simulink model "FullyConnectedMMG"  (R2020b)
settings: Solver=ode3  StartTime=0.0  StopTime=TimeS  FixedStep=Ts  RelTol=1e-3
values from neighbouring files (symbols this model uses):
  fr = 60    [MMG_Parameters.m]
  Lgs = 600e-6    (= 0.0006)    [MMG_Parameters.m]
  MaxWind = 18    [MMG_Parameters.m]
  MicroVol = 575    [MMG_Parameters.m]
  MinWind = 3    [MMG_Parameters.m]
  NomVol = 600    [MMG_Parameters.m]
  NomWind = 10    [MMG_Parameters.m]
  Pnombb = 400    [MMG_Parameters.m]
  PnomDG = 150e3    (= 150000)    [MMG_Parameters.m]
  PnomWT = 400e3    (= 400000)    [MMG_Parameters.m]
  Rgs = 20e-6    (= 2e-05)    [MMG_Parameters.m]
  RtCapM1 = (5.1)*1e-1    (= 0.51)    [MMG_Parameters.m]
  RtCapM2 = (5.1)*1e-1    (= 0.51)    [MMG_Parameters.m]
  SOC = [70,80,75,65]    [MMG_Parameters.m]
  Ts = 8e-4    (= 0.0008)    [MMG_Parameters.m]    (also in SolveMONO.m = 0.005)
  Vgrid = 25e3    (= 25000)    [MMG_Parameters.m]
  VMic = 575    [MMG_Parameters.m]
  Vs = 120e3    (= 120000)    [MMG_Parameters.m]
undefined symbols (not defined in the file or in its folder): DiscIntNeverNeededParam
libraries: powerlib x64, simulink x24, powerlib_meascontrol x16
(part 4 of 5)

== matlab function FullyConnectedMMG/Subsystem/Subsystem2/MATLAB Function ==
  settings: updateMethod=DISCRETE
  data: Hour input; xInput input; outGrid output; shMGs output; recMGs output; Flag output
 function [outGrid,shMGs,recMGs,Flag] = States(Hour,xInput)
%% Parameters For Objective Function %%
%%%%%%%%%%%%%%%%%%%%%%%%%%%%%%%%%%%%%%%
% The objective function in the second layer is established to improve costs in the entire MMG system -%
% The CEMS in this layer aims to minimize costs caused by power exchanged between MGs into 
% the MMG system and as well as power losses caused by transactions % 

% ********************** %
% The Objective Function %
% ********************** %
% f =  sum(Cg*(Pm^{Ug}(t) + Pm^{lossg}(t)) + Cexc(Pmj^{exc}(t) + Pmj^{lossMG}(t))

% Note: It is important to note that in this case we only need one RNN
% to solve the single-objective optimization problem. 

%%%%%%%%%%%%%%%%%%%%%%%%%%%%%%%%%%%%%%%%%%%%%%%
%% Call The Function That Containts The DPNN %%
%%%%%%%%%%%%%%%%%%%%%%%%%%%%%%%%%%%%%%%%%%%%%%%
% In this case, xInput are the references for power exchanged between the
% MGs and the grid established in the first layer by the NEMS  
% Hour, is the respective time slot.

numMGs = length(xInput);                        	% Number of MGs within the MMG system

%- Define the dimension of output variables -%
outGrid = zeros(numMGs,1); shMGs = zeros(numMGs,1);  recMGs = zeros(numMGs,1);  oErr = zeros(numMGs,1);  Flag = 0;

%- Call the main function to perform the optimization in the CEMS -%
[outGrid,shMGs,recMGs,oErr,Flag] = Optimization(xInput, Hour, numMGs);

%- Print information about optimization -%
    nMGs = (1:numMGs);
    status = cell(numMGs,1);
    
    for k=1:length(nMGs)
        if xInput(k) < 0
            status{k} = 'Surplus';
        else
            status{k} = 'Deficit';
        end
    end
    
    wkW = 1e-3;
    fprintf(' ------------------------------------------------- \n || Info about optimization in the second layer || \n ------------------------------------------------- \n');
    Table2 = table((wkW)*xInput,status,(wkW)*outGrid,(wkW)*shMGs,(wkW)*recMGs,oErr,...
                'VariableNames',{'| Ener. net |','| Status |','| Ener. Grid |','| Ener. shared |','|Ener. received |','| Error |' },'RowName',{'|| MG1 ||','|| MG2 ||'})
    fprintf('\n|| -o-o-o-o-o-o-o-o-o-o-o-o-o-o-o-o-o-o-o-o-o-o-o-o-o-o-o-o-o-o-o-o-o-o-o-o-o-o-o-o-o-o-o-o-o-o-o-o-o-o-o-o-o-o-o-o-o-o-o-o-o-o-o-o-o-o-o-o-o-o-o-o-o-o-o-o-o-o-o-o-o- ||');    
    
    %formatSpec = '|| MG %1.0f || Status: %s, EnergyNet: %4.2f, Grid: %4.2f, Sharing: %4.2f, Receiving: %4.2f, Error: %3.2f \n';
    %fprintf(' --------------------------------------- \n | Info of optimization in the second layer | \n --------------------------------------- \n');
    %for k=1:length(nMGs)
    %    if xInput(k) < 0
    %        status = "Sur";
    %    else
    %        status = "Def";
    %    end
    %    fprintf(formatSpec,nMGs(k),status,xInput(k),outGrid(k),shMGs(k),recMGs(k),oErr(k));
    %end
% fprintf('\n|| -o-o-o-o-o-o-o-o-o-o-o-o-o-o-o-o-o-o-o-o-o-o-o-o-o-o-o-o-o-o-o-o-o-o-o-o-o-o-o-o-o-o-o-o-o-o-o-o-o-o-o-o-o-o-o-o-o-o-o-o-o-o-o-o-o-o-o-o-o-o-o-o-o-o-o-o-o-o-o-o-o- ||');    

end

% %%%%%%%%%%%%%%%%%%%% %
%- Auxiliar Functions -%
% %%%%%%%%%%%%%%%%%%%% %

% **************************** %
%- Main Optimization Function -%
% **************************** %
function [oGrid,shMGs,recMGs,oErr,Flag] = Optimization(eInp,hr,nMG)
%%%%%%%%%%%%%%%%%
%% Some notes: %%
%%%%%%%%%%%%%%%%%
%%%%%%%%%%%%%%%%%%%%%%%%%%%%%%%%%%%%%%%%%%%%%%%%%%%%
%- This function will output two vectors, where:   %
%  oGrid = [Energy imp/exp from/to grid in MG_m];  %


%  oMGs = [Energy imp/exp from/to MGj in MG_m];    %
%  For m = 1,.., M.                                %

%  oGrid and oMGs are vectors of dimension 
% [nMG x 1], respectively. -%
%%%%%%%%%%%%%%%%%%%%%%%%%%%%%%%%%%%%%%%%%%%%%%%%%%%%

%- eInp = Energy statuts (Surplus/deficit energy in each MG) -%
    Auxv = zeros(nMG,1);                    % Auxiliar vector to check the status of energy in MGs (deficit/surplus)
    for i=1:nMG
        if eInp(i) < 0
            Auxv(i,1) = 1;                  % "1" Means that there exists surplus energy
        else
            Auxv(i,1) = 0;                 	% "0" Means that there exists deficit energy
        end
    end
 
    surVect = find(Auxv);                 	% Indixes of MGs with surplus energy 
    lenSur = length(surVect);            	% Number of MGs with surplus energy
    
    defVect = find(~Auxv);                 	% Indixes of MGs with deficit energy
    lenDef = length(defVect);            	% Number of MGs with deficit energy
    
%%%%%%%%%%%%%%%%%%%%%%%%%%%%%%%%%%%%%%%%%%%%%%%%%%%%%%%%%%%%%%%    
%- Perform theans Global Optimization If There Exist Conditions -%
%%%%%%%%%%%%%%%%%%%%%%%%%%%%%%%%%%%%%%%%%%%%%%%%%%%%%%%%%%%%%%%
    EnableGO = 0;                                   % Enable Global Optimization (1= Enable, 0 = Disable)
    %- Check that there exist one MG with surplus and 
    % other one with deficit energy.
    if (lenSur ~= 0 && lenDef ~= 0 && EnableGO ==1)       
    % Use neural netowrk function to perform the optimization %
        [outX,oErr] = NNfunc(surVect,defVect,eInp,nMG,hr);       
        oGrid = outX(:,1);
        shMGs = outX(:,2);
        recMGs = outX(:,3);
    else
        % Not perform the optimization because the conditions are not satisfied.
        oGrid = eInp;                                       
        shMGs = zeros(nMG,1);                               
        recMGs = zeros(nMG,1);
        
        oErr = (11.11)*ones(nMG,1);
    end   
    Flag = hr + 1;
end

% ************************* %
%- Neural Network Function -%
% ************************* %
function [xOpt,Error] = NNfunc(surVec,defVec,xEn,nMG,hour)
    %- Required parameters for neural networks -%
    nVar = 2;                                           % Number of desicion variables
    Ts = 5e-3;                                          % Step size for the solver
    Lamb = 6;                                           % Rate of convergence for the neural network (Workin: Lamb = ??);
    ite = 2500;              % 20000;                    % Max number of iterations to integrate the differential equations
    
    xOpt = [xEn,zeros(nMG,2)];                          % Establish the output vector
    
    %- Bounds for exchanged power in the MMG system -%     
    Mingrid = 0;                                        % (Kw/h)   Max power exported to the grid 
    Minsh = 0;                                          % (Kw/h)   Min power shared by an MG with surplus power
    
    %- Auxiliar variables -%
    shPower = zeros(length(surVec),nVar);               % Auxiliar vector to save the relation between MGs exchanging energy
    auxOpt = zeros(length(surVec),nVar);                % Auxiliar vector to save optimal values 
    
    Error = (11.11)*ones(nMG,1);                                % Auxiliar vector to observe the error produced during optimization
       
    % Maxgrid = (1e4)*150;                             	% kW/h   Max power imported from the grid
    
    %%%%%%%%%%%%%%%%%%%%%%%%%%%%%%%
    %- Main Loop of optimization -%
    %%%%%%%%%%%%%%%%%%%%%%%%%%%%%%%
    %- Select an MG with surplus energy and perform an optimization with
    % each MG with deficit of power. 
    for i=1:length(surVec)                         
        vecX = zeros(length(defVec),2);               	% Auxiliar vector of solutions
        costX = zeros(length(defVec),1);             	% Auxiliar vector of costs
        
        for j=1:length(defVec)
         	Maxgrid = abs(xEn(surVec(i)));          	% The Max power that can inject to the grid is the 
                                                        % total of surplus energy 
            
            Maxsh_rec = min(Maxgrid,xEn(defVec(j)));    % The max power received by a MG will be the min 
                                                        % between the surplus power of MGi and deficit power of MGj
            
            %- Establish the upper and lower bounds for decision variables -%                                            
            UpB = [Maxgrid;Maxsh_rec];                  % Upper bound
            LowB = [Mingrid;Minsh];                     % Lower bound
            % -------------------------------------------------------------- %
            %- Call objective function f(x) and its derivative in this layer %
            % ---------------------------------------------------------------% 
            [Func,gFunc] = ObjFunct(xEn,i,j,hour);   
            %- Variables used for the equality constraint -%
            A = [1,1];                                  % We have only two variable decisions:
                                                        % Energy shared
                                                        % with the grid and the energy shared with other MG
                                                        
            b = abs(xEn(surVec(i)));                    % In this case, we consider the energy shared with the grid 
                                                        % and with other MG j mustbe the same of surplus energy in MG i 

           	%- Initial value for decision variable x -%
          	Ic = abs(UpB(1))/2;
            % Iincr = 20;
            Iincr = abs(UpB(1))/15;
            
            x = [Ic-Iincr;Ic+Iincr];
            
            % x = [unifrnd(Mingrid,Maxgrid);unifrnd(Minsh,Maxsh_rec)]; 
            
            %- Check these conditions (Maybe are not necessary) -%
            counter = 1;
            condConv = true;
            
            %%%%%%%%%%%%%%%%%%%%%%%%%%%%%%%%%%
            %- Main loop of neural networks -%
            %%%%%%%%%%%%%%%%%%%%%%%%%%%%%%%%%%                     
            while condConv
                %%%%%%%%%%%%%%%%%%%%%%%%%%%%%%%%%%%%%%%%%%%%
                %- Structure of recurrent neural networks -%
                %%%%%%%%%%%%%%%%%%%%%%%%%%%%%%%%%%%%%%%%%%%%
                % ************************* %
              	% Structure of our approach %
              	% ************************* %
                sig = -(0.5)*ones(1,1);                             % Initial values for sigma 
                Px = zeros(length(x),1);                            % Auxiliar variable for the projection
                %- Gains used by the activation functions y and z %
                if hour == 14
                    k2 = 100;     % Original values
                    k1 = 85.5;    % Original values    
                elseif hour == 15
                    k2 = 100;     % Original values
                    k1 = 205.5;    % Original values    
                else
                    k2 = 100;
                    k1 = 65.5;  
                end

                %- Integrate the differential equations of neural networks -% 
                for it=1:ite                           	              
                    % Finite-Time Stabilizer (Lagrange Multiplier y)%
                    y = Stabilizer(UpB,LowB,k2,x);
                    % Finite-time sliding mode operator (Lagrange Multiplier z) %
                    z = SMOperator(UpB,LowB,k1,x,sig);    
                    %- Apply the projection -%
                  	for n = 1:length(x)
                        Px(n,1) = Pr(LowB(n),UpB(n),x(n));          	 
                    end
                    %- Dynamic for Recurrent Neural Network -%
                    dx = Lamb*(-gFunc(Px) + Px - x + A'*z + y);
                    %- Dynamic for variable related with the sliding surface -%
                    dsig = Lamb*(-A*gFunc(Px) + A*Px - A*x + A*A'*z + A*y); 
                    %- Integration of differential equations related to neural networks -%
                    tspan = [0 Ts];
                    [~,xout] = ode23(@(tx,xout) dx, tspan, x);
                    [~,sigout] = ode23(@(tz,sigout) dsig, tspan, sig);
                    %- Output variables of ODE -%
                    x = xout(end,:)';
                    sig = sigout(end,:);
                    %- Check the error obtained -%
                    if abs(sum(x) - b) < 0.5                %Work: 0.3
                        condConv = false;
                        break;
                    end
                end
             	counter = counter + 1;
                if counter > 4
                    condConv = false;
                end               
            end 
            vecX(j,:) = x';
            costX(j) = Func(x); 
        end
        
        % Select Solutions With Best Values (Minor Costs) %
        [~,Index] = min(costX);
        % Save The Relation Between There Exists a Exchanged Power
        shPower(i,:) = [surVec(i),defVec(Index)];
        % Save Optimal Values %
        auxOpt(i,:) = vecX(Index,:);
        % Determinate Errors;
        Error(surVec(i)) = abs(sum(auxOpt(i,:)) - abs(xEn(surVec(i))));
        % Modify Output Vector Of Exchanged Power %
        xOpt(surVec(i),1:2) = -vecX(Index,:);
        % xOpt(surVec(i),3) = 0;
        xOpt(defVec(Index),1) = xOpt(defVec(Index),1) - vecX(Index,2);
        %xOpt(defVec(Index),2) = 0;
        xOpt(defVec(Index),3) = vecX(Index,2);
        
        % Delete Used Indexes %
        % surVec(i) = [];
        defVec(Index) = [];
        if isempty(defVec)
            break;
        end
    end
end
   
% ******************** %
%- Objective Function -%
% ******************** %
function [Func,gFunc] = ObjFunct(eneVec,i,j,hr)
    %- Establish the cost of grid energy according the hour of the day -%
    peak = [(8:11),(16:21)];                % (Hr) Period of time for peak tariff category 
    plain = (12:15);                        % (Hr) Period of time for plain tariff category
    %   valley = [(1:7),(22:24)];          	% (Hr) Period of time for valley tariff category
    if ismember(hr,peak)
        % Peak tariff %
        Cgpur = 0.21;   %0.17               % (USD/Kwh) Cost of purchasing energy from the grid 
        Cgsell = 0.11;                      % (USD/kWh) Cost of selling energy to the grid
    elseif ismember(hr,plain)
       	% Plain tariff %
        Cgpur = 0.14;                       % (USD/Kwh) Cost of purchasing energy from the grid 
        Cgsell = 0.051;                     % (USD/kWh) Cost of selling energy to the grid
    else
        % Valley tariff % 
        Cgpur = 0.062;                      % (USD/Kwh) Cost of purchasing energy from the grid
        Cgsell = 0.039;                     % (USD/kWh) Cost of selling energy to the grid
    end  
    %- Check if energy will be purchased/sold from/to the grid -%
    if eneVec < 0   
        % Cg = Cgpur;                       % The MG is purchasing energy from the grid   
        sell = 0;
        Pur = 1;
    else
        %Cg = Cgsell;                       % The MG is sellig energy to the grid
        sell = 1;
        Pur = 0;
    end
    % Volatage in transmission lines %
    UMG = 575;                              % (V) voltage of the distribution lines in the MMG system
    % Cheeeeeeeeeeeeeeeeeeeeeeeeeeck this voltage %
    Ugrid = 575;                            % (V) voltage of the distribution lines between the MGs and the grid
    % AuxRgrid = [1.55,1.75,1.875,1.7];
    AuxRgrid = [3.1,3.15,3.705,2.5875];
    Rgrid = AuxRgrid(i);                    % (Ohms) Resistance of the distribution lines between MG i and the grid 
    %- Resistance in transmission lines among the MGs within the MMG system -%
    AuxRMGs = [ 1,   0.4,  0.1,  0.08;
            0.4,  1,   0.06, 0.05;
            0.1,  0.06, 1,   0.02;
            0.08, 0.05, 0.02, 1];
        
    RMGs = AuxRMGs(i,j);                    % Select the resistence of transmission lines between MGi and MGj
    %- Coeffcients costs (of sharing-receiving power among MGs) -%
    Csh = 0.005;        % 0.01;           	% (USD/Kwh) Cost of share (sell) energy with other MG
    Crec = 0.005;       % 0.01;            	% (USD/Kwh) Cost Of receieve (purchase) energy from other MG
    %%%%%%%%%%%%%%%%%%%%%%%%%%%%%%%%%%%%%%
    %% Objective function (in the CEMS) %%
    %%%%%%%%%%%%%%%%%%%%%%%%%%%%%%%%%%%%%%
    %- Objective Function -%
    Plossgrid = @(x) (x(1)^2)*(Rgrid/(Ugrid^2));
    PlossMG =   @(x) (x(2)^2)*(RMGs/(UMG^2));
    
    Func =  @(x) Pur*Cgpur*x(1) + sell*Cgsell*x(1) + Pur*Cgpur*Plossgrid(x) + sell*Cgsell*Plossgrid(x)...
                +Pur*Crec*x(2) + sell*Csh*x(2) + sell*Csh*PlossMG(x) + Pur*Crec*PlossMG(x);
    
    %- Gradient of objective optimization function -%
    gFunc = @(x) [Pur*Cgpur + sell*Cgsell + Pur*Cgpur*2*x(1)*(Rgrid/(Ugrid^2)) + sell*Cgsell*2*x(1)*(Rgrid/(Ugrid^2));
                  sell*Csh + Pur*Crec + sell*Csh*2*x(2)*(RMGs/(UMG^2)) + sell*Cgsell*2*x(2)*(RMGs/(UMG^2))];   

    % Check if the output values of these functions coincide with the above functions %
              
    % Func1 =  @(x) Pur*Cgpur*x(1) + sell*Cgsell*x(1) + Pur*Cgpur*(x(1)^2)*(Rgrid/(Ugrid^2)) + sell*Cgsell*(x(1)^2)*(Rgrid/(Ugrid^2))...
    %            + sell*Csh*x(2) + Pur*Crec*x(2) + sell*Csh*(x(2)^2)*(RMGs/(UMG^2)) + Pur*Crec*(x(2)^2)*(RMGs/(UMG^2));
              
    % gFunc = @(x) [Pur*Cgpur + sell*Cgsell + Pur*Cgpur*2*x(1)*(Rgrid/(Ugrid^2)) + sell*Cgsell*2*x(1)*(Rgrid/(Ugrid^2));
    %              sell*Csh + Pur*Crec + sell*Csh*2*x(2)*(RMGs/(UMG^2)) + sell*Cgsell*2*x(2)*(RMGs/(UMG^2))];                 

%{
    % Objective Function %
    Func =  @(x) fExp*fEimp*Cgpur*x(1) + fExp*fEimp*Cgsell*x(1) + Closs*(x(1)^2)*(Rgrid/(Ugrid^2))...
                + fExp*fEimp*Csh*x(2) + fExp*fEimp*Crec*x(2) + Closs*(x(2)^2)*(RMGs/(UMG^2));
    
    %- Gradient of Objective Optimization Function %
    gFunc = @(x) [fExp*fEimp*Cgpur + fExp*fEimp*Cgsell + 2*Closs*x(1)*(Rgrid/(Ugrid^2));
                  fExp*fEimp*Csh + fExp*fEimp*Crec + 2*Closs*x(2)*(RMGs/(UMG^2))];
%}              
end

% ********************************** %
%- Function to apply the projection -%
% ********************************** %
function y = Pr(Lbx, Ubx, xin)
    y = 0;
    idx1 = xin <= Lbx;
    y(idx1) = Lbx;
    idx2 = xin >= Ubx;
    y(idx2) = Ubx;
    y(~(idx1 | idx2)) = xin;
end

% ********************************************************************** %
%- Finite Time Stabilizer Function (Used to reach the bound constraints)-%
% ********************************************************************** %
function Outy = Stabilizer(Ubx,Lbx,k,eta)
    % Auxiliar variables %
    Outy = zeros(length(eta),1); 
    xl = norm(eta - Lbx);  
    xh = norm(eta - Ubx);
    % Select Case %
    for i = 1:length(eta)
        if eta(i) < Lbx(i)          % x < l
            Outy(i,1) = -k*((eta(i) - Lbx(i))/xl);
        elseif  eta(i) > Ubx(i)     % x > h
            Outy(i,1) = -k*((eta(i) - Ubx(i))/xh);
        else
            Outy(i,1) = 0;
        end
    end
end

% *************************************************************** %
%- Finite time sliding mode operator:                             % 
% (Used to reach the sliding surface inside the bound constraints %
% *************************************************************** %
function Outz = SMOperator(Ubx,Lbx,k,eta,sig)
  	% Auxiliar variables %
    % Outz = zeros(length(sig),1);    
    % Check Bounds and Select Case %
    if eta > Ubx           
        Outz = zeros(length(sig),1);
    elseif eta < Lbx
        Outz = zeros(length(sig),1);
    else
        Outz = -k*(sig/norm(sig));     % l < x < h
    end
        
end

% **************** %
%- Delay Function -%
% **************** % 
%{
function [x,z] = delayfnc(ux,uz)
% Unit delay implementation that maps to a register in hardware %
% Initial Conditions %
ICx = [0;0]; ICz = 0;
persistent u_x1 u_z1;
    if isempty(u_x1)
        % defines initial value driven by unit delay at time step 0
        u_x1 = cast(ICx, 'like', ux);
        u_z1 = cast(ICz, 'like', uz);
    end
% return delayed input from last sample time hit
x = u_x1; z = u_z1;
% store the current input
u_x1 = ux; u_z1 = uz;
end
%}

% Structure of neural network proposed by Xia in:
% An extended projection neural network for constraint optimization
%{
%- Initial States -%
xS1 = [unifrnd(Mingrid,Maxgrid);unifrnd(Minsh,Maxsh_rec)];               % Initial Decisition State x
zS1 = (1e-1);                                      	% Initial Hidden State z
x = xS1;  z = zS1;
Ps1 = zeros(length(x),1);                          	% Auxiliar variable for the projection

delayfnc([0;0],0);                                      % Clear Delay Function

for it=1:ite                                         	% Number of Iterations For Convergence % (605);
    Ta = x - gFunc(x) + A'*z;
        for n = 1:length(Ta)
            Ps1(n,1) = piecewisex(LowB(n),UpB(n),Ta(n));       	% Apply The Projection %
        end
    % Discrete Neural Networks (Using Euler Method) %
    dx = x + Ts*(Lamb*(-x + Ps1));                             	% x State
    dz = z + Ts*(Lamb*(-A*x + b));                             	% z State
    [x,z] = delayfnc(dx,dz);                              	    % Function Delay %
    if abs(sum(x) - b) < 0.5                %Work: 0.3
        condConv = false;
        break;
    end
end
%}

== matlab function FullyConnectedMMG/Subsystem/Subsystem/MATLAB Function ==
  settings: updateMethod=DISCRETE
  data: hr input; CMG1 output; CMG2 output; CostMMG output; xMG1 input; xMG2 input; PLMMG output; SOCMMG input
function [CMG1,CMG2,CostMMG,PLMMG] = fcn(hr,xMG1,xMG2,SOCMMG)

%%%%%%%%%%%%%%%%%%%%%%%%%%%%%%%%%%%%%
%% Costs Of MGs In The First Layer %%
%%%%%%%%%%%%%%%%%%%%%%%%%%%%%%%%%%%%%
% PgridMG1 = xMG1(1); PpvMG1 = xMG1(4); PwtMG1 = xMG1(5); PbbMG1 = xMG1(6); PdgMG1 = xMG1(7);
    % ************** % 
    %- Costs in MG1 -%
    % ************** %
    Cg = zeros(1,2);
	% Operating and Enviromental Costs %
    [OcM1,EcM1,Cg(1),GCMG1,EmMG1] = EvalCost(hr,xMG1,SOCMMG(1)); 

    % ************** % 
    %- Costs in MG2 -%
    % ************** %
	% Operating and Enviromental Costs %
    [OcM2,EcM2,Cg(2),GCMG2,EmMG2] = EvalCost(hr,xMG2,SOCMMG(2)); 
   
    %%%%%%%%%%%%%%%%%%%%%%%%%%%%%%%%%%%%%%
    %% Costs Of MGs In The Second Layer %%
    %%%%%%%%%%%%%%%%%%%%%%%%%%%%%%%%%%%%%%    
  	% Volatages in Transmission Lines %
    UMG = 575;                              % (V) voltage of the distribution line in the Cooperative Scheme
    Ugrid = 575;                            % (V) voltage of the distribution line between MG and the main grid
    
    % Resistance in Transmission Lines %
    RgMG1 = 3.1;                             % (Ohms) Resistance of the distribution line between MG 1 and the main grid 
    RgMG2 = 3.15;                            % (Ohms) Resistance of the distribution line between MG 2 and the main grid
    RgMG3 = 3.705;                           % (Ohms) Resistance of the distribution line between MG 3 and the main grid
    RgMG4 = 2.58;                            % (Ohms) Resistance of the distribution line between MG 4 and the main grid
    
    %- Check The MGs Wich Are Sharing Power -%
    shP = [xMG1(2);xMG2(2)];
    recP = [xMG1(3);xMG2(3)];
    
    %- Check MGs That Are Sharing Power -%
    [auxSh,~]  = find(shP);
    [auxRec,~] = find(recP);
    
    %- Auxiliar Vector To Save Index Of MGs That Are Sharing Energy -%
    auxIndex = zeros(length(auxSh),2);
    
    for j=1:length(auxSh)
       for k=1:length(auxRec)
            if abs(shP(auxSh(j))) == abs(recP(auxRec(k)))
                auxIndex(j,:) = [auxSh(j),auxRec(k)];
            end
       end
    end
     
    %- Resistance in Transmission Among The MGs Into The MMG System -%
    AuxRMGs = [ 1,    0.4,  0.1,  0.08;
                0.4,  1,    0.06, 0.05;
                0.1,  0.06, 1,    0.02;
                0.08, 0.05, 0.02, 1];
    
    %- Only Assing Resistences That are Sharing Energy -%
    RMGs = zeros(4,1);
    
    [S,~] = size(auxIndex);
    for j=1:S
        RMGs(auxIndex(j,1)) = AuxRMGs(auxIndex(j,1),auxIndex(j,2));
    end
    
    % Coeffcients Costs %
    Csh = 0.005;% 0.01;                                 % USD/Kwh Cost of Share Energy With Other MG
    % Crec = 0.005; % 0.01;                                % USD/Kwh Cost Of Receieve Energy From Other MG
    
    Floss = 20;
    CFloss = 0.6;
    
    % Global Cost in MG1 %
    PL_MG1grid = Floss*(xMG1(1)^2)*(RgMG1/(Ugrid^2));
    PL_MG1mg = Floss* (xMG1(2)^2)*(RMGs(1)/(UMG^2));
    
    ClossMG1 = (CFloss+Cg(1))*PL_MG1grid + (CFloss+Csh)*PL_MG1mg; % Cost Due of Power Transactions
    % gcMG1 = ClossMG1; % + Csh*xMG1(2) + Crec*xMG1(3);
    
    % Global Cost in MG2 %
    PL_MG2grid = Floss*(xMG2(1)^2)*(RgMG2/(Ugrid^2));
    PL_MG2mg = Floss*(xMG2(2)^2)*(RMGs(2)/(UMG^2));
    
    ClossMG2 = (CFloss+Cg(2))*PL_MG2grid + (CFloss+Csh)*PL_MG2mg; 
    % gcMG2 = ClossMG2; % + Csh*xMG2(2) + Crec*xMG2(3);
    
    % Global Cost in MG3 %
    % PL_MG3grid = Floss*(xMG3(1)^2)*(RgMG3/(Ugrid^2));
    % PL_MG3mg = Floss*(xMG3(2)^2)*(RMGs(3)/(UMG^2));
    
    % ClossMG3 = (CFloss+Cg(3))*PL_MG3grid + (CFloss+Csh)*PL_MG3mg;
    % gcMG3 =  ClossMG3; % + Csh*xMG3(2) + Crec*xMG3(3);
    
    % Global Cost in MG4 %
    % PL_MG4grid = Floss*(xMG4(1)^2)*(RgMG4/(Ugrid^2));
    % PL_MG4mg = Floss*(xMG4(2)^2)*(RMGs(4)/(UMG^2));
    
	% ClossMG4 = (CFloss+Cg(4))*PL_MG4grid + (CFloss+Csh)*PL_MG4mg;
    % gcMG4 =  ClossMG4; % + Csh*xMG4(2) + Crec*xMG4(3);
    
    
	PLMG2 = PL_MG2grid + PL_MG2mg;
    PLMG1 = PL_MG1grid + PL_MG1mg;
    % PLMG3 = PL_MG3grid + PL_MG3mg;
    % PLMG4 = PL_MG4grid + PL_MG4mg;
    
%%%%%%%%%%%%%%%%%%%%%%%%%%%%%%%%%%%%%%%%%%%%%%%%%%%%%%%%%%%%%%%%%%%%%%%%    
%% Final Costs Of Every MG (Including The First And The Second Layer) %%
%%%%%%%%%%%%%%%%%%%%%%%%%%%%%%%%%%%%%%%%%%%%%%%%%%%%%%%%%%%%%%%%%%%%%%%%
  
    % Economic and Environmental Costs Of Each MG %
    CMG1 = [OcM1;EcM1;GCMG1;ClossMG1];
    CMG2 = [OcM2;EcM2;GCMG2;ClossMG2];
    % CMG3 = [OcM3;EcM3;GCMG3;ClossMG3];
    % CMG4 = [OcM4;EcM4;GCMG4;ClossMG4];

	% Total Local Costs In MGs%
	Ocost = OcM1 + OcM2;                          % Operating Costs In The Entire MMG System
    Ecost = EcM1 + EcM2;                          % Environmental Costs In The Entire MMG System
	
    % Total Cost In The MMG System by Power losses %
    Losscost = ClossMG1 + ClossMG2;      	% Costs Due Power Loss and Energy transactions (MGs-Grid & MGs-MGs)
    
    % Total Emission of CO2 %
    TotalEm = EmMG1 + EmMG2;
    
    % Total Costs In The Entire MMG System %
    Totalcost = Ocost + Ecost + Losscost;                    
    
    % Costs due to Power Loss in MGs %
    % CostPL = [ClossMG1;ClossMG2;ClossMG3;CstlossMG4];  % Costs Caused Only By Power loss in MGs
    
    % Power Loss in MGs %
    TPLMMG = PLMG1+PLMG2;
    PLMMG = TPLMMG;              % (kW/h)
    
    % Establish Output Costs %
    CostMMG = [Ocost;Ecost;TotalEm;Totalcost];    
    
end


function [OMCost,EnvCost,Cg,GridCost,Emissions] = EvalCost(hr,xMG,SOC)
    %- Costs of Grid Energy -%
        peak = [(8:11),(16:21)];                % (Hr) Period Range of Peak Tariff Category 
        plain = (12:15);                        % (Hr) Period Range of Peak Tariff Category
        
    %   valley = [(1:7),(22:24)];          	% (Hr) Period Range of Peak Tariff Category
        if ismember(hr,peak)
            % Peak Tariff %
            Cgpur = 0.21;                       % (USD/Kwh) Cost of Purchasing Energy From The Grid 
            Cgsell = -0.11;                     % (USD/Kwh) (It is negative because the MG1 is receiving an incoming from selling energy)          
        elseif ismember(hr,plain)
            % Plain Tariff %
            Cgpur = 0.14;                       % (USD/Kwh) Cost of Purchasing Energy From The Grid 
            Cgsell = -0.051;                    % (USD/Kwh) (It is negative because the MG1 is receiving an incoming from selling energy)          
        else
            % Valley Tariff % 
            Cgpur = 0.062;                      % (USD/Kwh) Cost of Purchasing Energy From The Grid
            Cgsell = -0.039;                    % (USD/Kwh) (It is negative because the MG1 is receiving an incoming from selling energy)          
        end

    % Emission Values Of CO2 For The Main Grid %
        co2g = 388.55;                          % g/Kwh (CO2)
        % so2g = 1.4; 
        % noxg = 1.3;


        Eco2 = 0.00287;                         % USD/Kg Cost by Penalization by CO2 Emissions  

        % bgg = sum(betag.*gamma);
        % bgg = co2g*Eco2;    


    %- Coeffcients Costs Of Non-Dispatchable DERs -%
        Cwt = 0.0296;                           % USD/Kwh   Wind Turbine Cost Generation
        Cpv = 0.0096;                           % USD/Kwh   PV Panel Cost Generation

    %- Coeffcients Costs of Battery Bank -%    
        % Linear Form %
        % Cbb = 0.082; %0.0648;                 % USD/Kwh   Battery Bank Cost Generation

        % Quadratic From %
        % ("Values Obtained from Paper: Multiagent-Based Optimal Microgrid Control
        % Using Fully Distributed Diffusion Strategy")
        aBBc = 11e-11; 
        bBBc = 8e-5;  
        cBBc = 1;      % 

        om = 1;     % 3

        Pbbmax = 400e3;                                     % Maximum Charge or Discharge rate of the battery

        % Cost of internal power trading between MGs %
        Csh = -0.005;        % 0.01;                         % USD/Kwh Cost of Share Energy With Other MG
        Crec = 0.005;       % 0.01;                     	% USD/Kwh Cost Of Receieve Energy From Other MG
    
        %- Coefficients Cost Of Diesel Generator -%   
        % Linear Form %
        % Paramaters obtained from paper: ("Efficient Energy Management of
        % Renewable Resources in Microgrids") 
        % Cdg = 0.024;                            % USD/Kwh   Diesel Generator Cost Generation          
        % Cfuel = 1.2;                            % USD/L Unit price of diesel
        % a = 0.0001;                             
        % b = 0.0438;                             
        % c = 0.3;

       % Emissions and Enviromental Vaule Of Diesel Generator %
        % co2 = 232.01;                           % g/Kwh  (CO2) Carbono Dioxide   
        % so2 = 0.464;                            % g/Kwh  (SO2) Sulfur Dioxide    
        % nox = 4.331;                            % g/Kwh  (NOx) Nitrogen Dioxide  
        % co = 2.32;                              % g/Kwh  (CO)  Carbon Oxide      


        % Eso2 = 0.75;                            % USD/kg  (SO2)  
        % Enox = 1;                               % USD/kg  (NOx) 
        % Eco = 0.125;                            % USD/kg  (CO) 
        % gamma = [Eco2;Eso2;Enox];

        % beta = [co2;so2;nox]; 
        % bg = beta.*gamma; 


        %- Quadratic form for Diesel Generator -%
        % Operating Cost Values Obtained from the paper: ("Primal dual interior point algorithm for...") %
        aDEc = 0.0547;
        bDEc = 1.7362;
        cDEc = 3.2456;

        % Environmenatl values Obtained from the Paper: ("Primal dual interior
        % point algorithm for...") 
        aDEe = 28.1444;
        bDEe = 1.7228;
        cDEe = 0.0017;

        % Check If Energy Will Be Purchased/Sold From/To The Grid    
            if xMG(1) < 0   
                Cg = Cgsell;                 % Cost of Selling Energy To The Grid
                AuxgE = 0;                   % (USD/Kg) Cost Of Emissions Due to Selling Energy To The Main Graid  
            else
                Cg = Cgpur;                  % Cost of Purchasing Energy From The Grid
                AuxgE = co2g;                 % (USD/Kg) Cost Of Emissions Due to Purchasing Energy From The Main Graid
            end
            
        % PgridMG = xMG(1); 
        % PpvMG = xMG(4); 
        % PwtMG = xMG(5); 
        % PbbMG = xMG(6); 
        % PdgMG = xMG(7);
        
        %Operating Cost %
        OMCost = aBBc*(xMG(6) + om*Pbbmax*(1-(SOC/100)))^2 + bBBc*(xMG(6) + om*Pbbmax*(1-(SOC/100))) + cBBc + ...
                    aDEc*(xMG(7)^2) + bDEc*xMG(7) + cDEc + Cg*xMG(1) + ...
                    Cwt*xMG(5) + Cpv*xMG(4) + Csh*xMG(2) + Crec*xMG(3);
          
        % Enviromental Cost %
        EnvCost = Eco2*(aDEe*xMG(7)^2 + bDEe*xMG(7) + cDEe + AuxgE*xMG(1));
        
        % Only the cost of the grid %
        GridCost = Cg*xMG(1) + Eco2*AuxgE*xMG(1);
        
        % Emissions of Pollutant CO2 (Grid and DGs) (Kg/kW)%
        Emissions = aDEe*xMG(7)^2 + bDEe*xMG(7) + cDEe + AuxgE*xMG(1);
end
